simulink model "example2"  (R2014a)
settings: Solver=ode45  StartTime=0.0  StopTime=10.0  RelTol=1e-3
settings Model: Creator=Радион  LastModifiedBy=Радион
settings DebuggingCC: SolverPrmCheckMsg=none

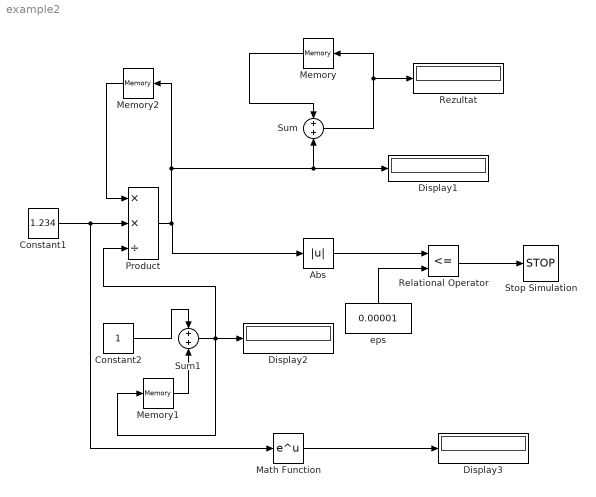
== system example2 ==
  Abs : Abs
  Constant1 : Constant  Value=1.234
  Constant2 : Constant
  Display1 : Display
  Display2 : Display
  Display3 : Display
  Math Function : Math  SaturateOnIntegerOverflow=on
  Memory : Memory  X0=1
  Memory1 : Memory
  Memory2 : Memory  X0=1
  Product : Product  Inputs=**/
  Relational Operator : RelationalOperator  Operator=<=  OutDataTypeStr=boolean
  Rezultat : Display
  Stop Simulation : Stop
  Sum : Sum  Inputs=+|+
  Sum1 : Sum  Inputs=+|+
  "eps " : Constant  Value=0.00001
  wires:
  Relational Operator/1 -> Stop Simulation/1
  "eps "/1 -> Relational Operator/2
  Math Function/1 -> Display3/1
  Constant1/1 -> Math Function/1, Product/2
  Constant2/1 -> Sum1/1
  Sum1/1 -> Memory1/1, Product/3, Display2/1
  Memory1/1 -> Sum1/2
  Memory2/1 -> Product/1
  Product/1 -> Display1/1, Sum/2, Memory2/1, Abs/1
  Abs/1 -> Relational Operator/1
  Sum/1 -> Memory/1, Rezultat/1
  Memory/1 -> Sum/1
